simulink model "Steering_model"  (R2018a)
settings: Solver=VariableStepAuto  StartTime=0.0  StopTime=simStopTime  RelTol=1e-3
PostLoadFcn:
  | helperLKASetUp
undefined symbols (not defined in the file or in its folder): lr, m, v0_ego, yaw0_ego
libraries: autolibshared x1
settings Model: Creator=The MathWorks, Inc.  LastModifiedBy=Emma
settings DebuggingCC: ParameterPrecisionLossMsg=none
settings HardwareCC: ProdLongLongMode=on

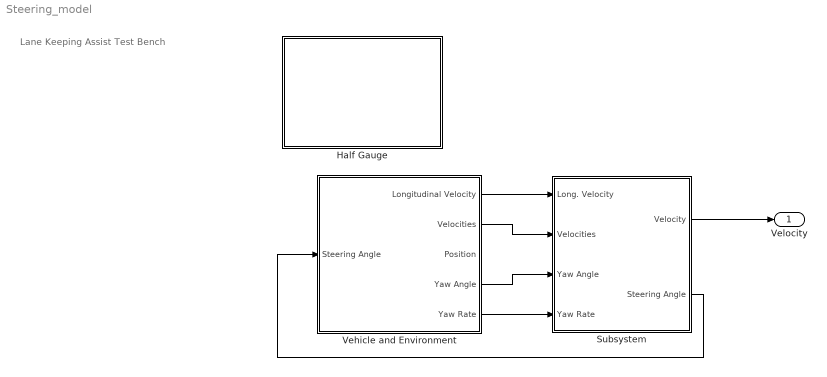
== system Steering_model ==
  note: Lane Keeping Assist Test Bench
  Half Gauge : Subsystem  DialogController=hmiCreateDDGDialog  IsWebBlock=on  mask(MWDashboardBlock){webBlockId=6cf1674e-b414-4085-9d76-7667875c1d24, webBlockType=semicirculargauge, ShowInLibBrowser=on, ShowInitialText=on, HMISrcModelName=Steering_model}
      mask prompts: webBlockId "WebBlock Id"; webBlockType "WebBlock Type"; HMISrcModelName "Source Model"
      mask help: SimulinkHMI:dialogs:SemicircularGaugeDialogDesc
      mask Help: helpview([docroot '/mapfiles/simulink.map'], 'hmi_half_gauge')
      mask Display:
      | if strcmp(get_param(bdroot(gcb),'BlockDiagramType'), 'library')
      |     image([(matlabroot) '/toolbox/simulink/hmi/icons/SemicircularGauge.png']);
      | end
  Subsystem : Subsystem
  Vehicle and Environment : Subsystem
  Velocity : Outport
  wires:
  Vehicle and Environment/1(Longitudinal Velocity) -> Subsystem/1(Long. Velocity)
  Vehicle and Environment/2(Velocities) -> Subsystem/2(Velocities)
  Vehicle and Environment/4(Yaw Angle) -> Subsystem/3(Yaw Angle)
  Vehicle and Environment/5(Yaw Rate) -> Subsystem/4(Yaw Rate)
  Subsystem/2(Steering Angle) -> Vehicle and Environment/1(Steering Angle)
  Subsystem/1(Velocity) -> Velocity/1

== system Steering_model/Half Gauge ==

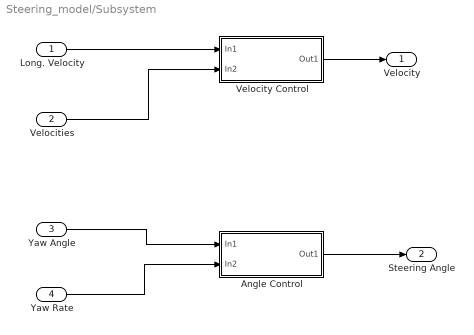
== system Steering_model/Subsystem ==
  Long. Velocity : Inport
  Velocities : Inport  Port=2
  Yaw Angle : Inport  Port=3
  Yaw Rate : Inport  Port=4
  Angle Control : Subsystem
  Velocity Control : Subsystem
  Velocity : Outport
  Steering Angle : Outport  Port=2
  wires:
  Long. Velocity/1 -> Velocity Control/1(In1)
  Velocity Control/1(Out1) -> Velocity/1
  Velocities/1 -> Velocity Control/2(In2)
  Yaw Angle/1 -> Angle Control/1(In1)
  Yaw Rate/1 -> Angle Control/2(In2)
  Angle Control/1(Out1) -> Steering Angle/1

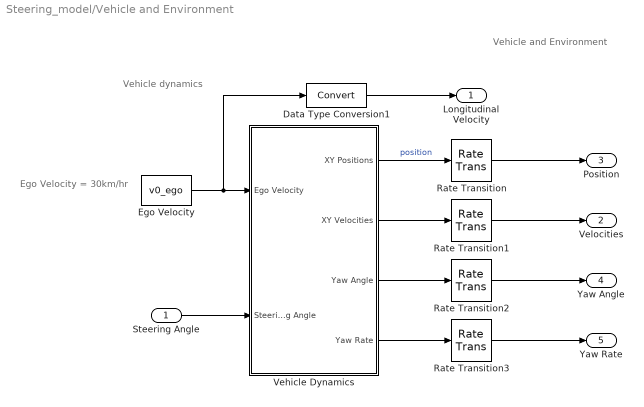
== system Steering_model/Vehicle and Environment ==
  note: Ego Velocity = 30km/hr
  note: Vehicle dynamics
  note: Vehicle and Environment
  Steering Angle : Inport  Unit=rad
  Data Type Conversion1 : DataTypeConversion
  Ego Velocity : Constant  Value=v0_ego
  Rate Transition{,1..3} (4 alike) : RateTransition  OutPortSampleTime=Ts
  Vehicle Dynamics : Subsystem  VariantControl=VariantVDBS
  Longitudinal Velocity : Outport  OutDataTypeStr=single  Unit=m/s
  Velocities : Outport  Port=2
  Position : Outport  Port=3
  Yaw Angle : Outport  Port=4
  Yaw Rate : Outport  Port=5
  wires:
  Ego Velocity/1 -> Data Type Conversion1/1, Vehicle Dynamics/1(Ego Velocity)
  Vehicle Dynamics/2(XY Velocities) -> Rate Transition1/1
  Vehicle Dynamics/3(Yaw Angle) -> Rate Transition2/1
  Vehicle Dynamics/4(Yaw Rate) -> Rate Transition3/1
  Vehicle Dynamics/1(XY Positions) -> Rate Transition/1  "position"
  Steering Angle/1 -> Vehicle Dynamics/2(Steering Angle)
  Data Type Conversion1/1 -> Longitudinal Velocity/1
  Rate Transition/1 -> Position/1
  Rate Transition1/1 -> Velocities/1
  Rate Transition2/1 -> Yaw Angle/1
  Rate Transition3/1 -> Yaw Rate/1

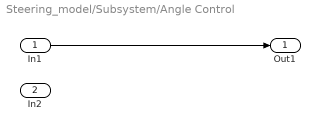
== system Steering_model/Subsystem/Angle Control ==
  In1 : Inport
  In2 : Inport  Port=2
  Out1 : Outport
  wires:
  In1/1 -> Out1/1

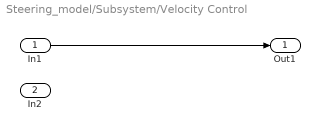
== system Steering_model/Subsystem/Velocity Control ==
  In1 : Inport
  In2 : Inport  Port=2
  Out1 : Outport
  wires:
  In1/1 -> Out1/1

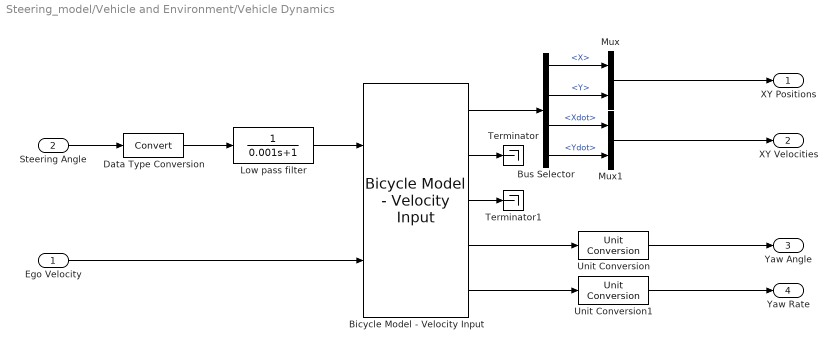
== system Steering_model/Vehicle and Environment/Vehicle Dynamics ==
  Ego Velocity : Inport
  Steering Angle : Inport  Port=2
  Bicycle Model - Velocity Input : autolibshared/Bicycle Model - Velocity Input  trackMode=Single (bicycle)  inputMode=External longitudinal forces  frontSteerMode=on  rearSteerMode=off  windMode=off  muMode=off  extFMode=off  extMMode=off  aMode=3  NF=2  NR=2  m=m  a=lf  b=lr  h=0.35  X_o=x0_ego  xdot_o=0  CalphaMode=off  sigmaMode=on  w=[1.4,1.4]  Cy_f=Cf  Cy_r=Cr  sigma_f=.1  sigma_r=.1  alpha_f_brk=[-.1 .1]  Cy_f_data=[-9e3 9e3]  alpha_r_brk=[-.1 .1]  Cy_r_data=[-9e3 9e3]  Y_o=y0_ego  ydot_o=0  Izz=Iz  psi_o=yaw0_ego*pi/180  r_o=0  Af=2  Cd=.3  Cl=.1  Cpm=.1  beta_w=[0:0.01:0.3]  Cs=[0:0.03:0.9]  Cym=[0:0.01:0.3]  Pabs=101325  Tair=273  g=9.81  mu=1  xdot_tol=.01  Fznom=5000  Fxtire_sat=1e6  Fytire_sat=1e6
      settings: SourceProductName=Powertrain Blockset  SourceProductBaseCode=PW
  Bus Selector : BusSelector  OutputSignals=InertFrm.FrntAxl.Disp.X,InertFrm.FrntAxl.Disp.Y,InertFrm.FrntAxl.Vel.Xdot,InertFrm.FrntAxl.Vel.Ydot
  Data Type Conversion : DataTypeConversion
  Low pass filter : TransferFcn  Denominator=[0.001 1]
  Mux : Mux  Inputs=2
  Mux1 : Mux  Inputs=2
  Terminator : Terminator
  Terminator1 : Terminator
  Unit Conversion : UnitConversion  OutputType=Inherit: Inherit via back propagation
  Unit Conversion1 : UnitConversion  OutputType=Inherit: Inherit via back propagation
  XY Positions : Outport  Unit=m
  XY Velocities : Outport  Port=2  Unit=m/s
  Yaw Angle : Outport  Port=3  Unit=deg
  Yaw Rate : Outport  Port=4  Unit=degree/s
  wires:
  Mux/1 -> XY Positions/1
  Mux1/1 -> XY Velocities/1
  Unit Conversion1/1 -> Yaw Rate/1
  Unit Conversion/1 -> Yaw Angle/1
  Ego Velocity/1 -> Bicycle Model - Velocity Input/2
  Bicycle Model - Velocity Input/1 -> Bus Selector/1
  Bicycle Model - Velocity Input/2 -> Terminator/1
  Bicycle Model - Velocity Input/3 -> Terminator1/1
  Bicycle Model - Velocity Input/4 -> Unit Conversion/1
  Bicycle Model - Velocity Input/5 -> Unit Conversion1/1
  Bus Selector/1 -> Mux/1  "<X>"
  Bus Selector/2 -> Mux/2  "<Y>"
  Bus Selector/3 -> Mux1/1  "<Xdot>"
  Bus Selector/4 -> Mux1/2  "<Ydot>"
  Data Type Conversion/1 -> Low pass filter/1
  Steering Angle/1 -> Data Type Conversion/1
  Low pass filter/1 -> Bicycle Model - Velocity Input/1
